simulink model "wing_landing_gear"  (R2015a)
settings: Solver=ode45  StartTime=0  StopTime=10  RelTol=1e-4  AbsTol=1e-4
model workspace (MAT data in the model file):
  grey = [0.5 0.5 0.5]
  lgrey = [0.7 0.7 0.7]
  dgrey = [0.3 0.3 0.3]
  ddgrey = [0.15 0.15 0.15]
  rho_alum = 2700
undefined symbols (not defined in the file): sigbuilder_block, X, Y, Z
libraries: sm_lib x59, sm_wing_landing_gear_lib x45, nesl_utility x7, simulink x2
(part 3 of 3)

== system wing_landing_gear/Wing Landing Gear/Main Column/Main Column/Spherical Cup and Holder/Cup ==
  Base-Center Transform : sm_lib/Frames and Transforms/Rigid Transform  TranslationMethod=StandardAxis  TranslationLengthUnit=cm  TranslationStandardAxis=+Z  TranslationStandardOffset=Ro  TranslationCartesianOffset=[0 0 0]  TranslationROffset=[]  TranslationROffsetUnits=m  TranslationZOffset=[]  TranslationZOffsetUnits=m  TranslationThetaOffset=[]  TranslationThetaOffsetUnits=deg  RotationMethod=None  RotationAngleUnits=deg  RotationStandardAxis=+X  RotationAngle=[]  RotationArbitraryAxis=[]  FollAlignAxisA=+X  BaseAlignAxisA=+Y  FollAlignAxisB=+Y  BaseAlignAxisB=+Z  RotationMatrix=[1 0 0; 0 1 0; 0 0 1]  BlockFunction=simmechanics.library.frames_transforms.rigid_transform
  Center-Strip A Transform : sm_lib/Frames and Transforms/Rigid Transform  TranslationMethod=None  TranslationLengthUnit=m  TranslationStandardAxis=+X  TranslationStandardOffset=0  TranslationCartesianOffset=[0 0 0]  TranslationROffset=[]  TranslationROffsetUnits=m  TranslationZOffset=[]  TranslationZOffsetUnits=m  TranslationThetaOffset=[]  TranslationThetaOffsetUnits=deg  RotationMethod=AlignedAxes  RotationAngleUnits=deg  RotationStandardAxis=+X  RotationAngle=[]  RotationArbitraryAxis=[]  FollAlignAxisA=+Y  BaseAlignAxisA=+Z  FollAlignAxisB=+Z  BaseAlignAxisB=-Y  RotationMatrix=[1 0 0; 0 1 0; 0 0 1]  BlockFunction=simmechanics.library.frames_transforms.rigid_transform
  Center-Strip B Transform : sm_lib/Frames and Transforms/Rigid Transform  TranslationMethod=None  TranslationLengthUnit=m  TranslationStandardAxis=+X  TranslationStandardOffset=0  TranslationCartesianOffset=[0 0 0]  TranslationROffset=[]  TranslationROffsetUnits=m  TranslationZOffset=[]  TranslationZOffsetUnits=m  TranslationThetaOffset=[]  TranslationThetaOffsetUnits=deg  RotationMethod=AlignedAxes  RotationAngleUnits=deg  RotationStandardAxis=+X  RotationAngle=[]  RotationArbitraryAxis=[]  FollAlignAxisA=+Z  BaseAlignAxisA=+X  FollAlignAxisB=+Y  BaseAlignAxisB=+Z  RotationMatrix=[1 0 0; 0 1 0; 0 0 1]  BlockFunction=simmechanics.library.frames_transforms.rigid_transform
  Cup Strip A : sm_lib/Body Elements/Solid  InertiaType=CalculateFromGeometry  Mass=[]  MassUnits=kg  CenterOfMass=[]  CenterOfMassUnits=m  MomentsOfInertia=[]  MomentsOfInertiaUnits=kg*m^2  ProductsOfInertia=[]  ProductsOfInertiaUnits=kg*m^2  DensityBased=on  Density=rho  DensityUnits=kg/(m^3)  GraphicType=FromGeometry  MarkerShape=Sphere  MarkerSize=10  MarkerSizeUnits=m  GraphicVisPropType=SimpleVisualProperties  GraphicDiffuseColor=Cc  GraphicSpecularColor=[0.8 0.8 0.8 1.0]  GraphicAmbientColor=[0.5 0.0 0.0 1.0]  GraphicEmissiveColor=[0.0 0.0 0.0 1.0]  GraphicShininess=64.0  GraphicOpacity=1  GeometryShape=GeneralExtrusion  RectangleSize=[]  RectangleSizeUnits=m  BrickDimensions=[]  BrickDimensionUnits=m  CylinderRadius=0.5  CylinderRadiusUnits=m  CylinderLength=1  CylinderLengthUnits=m  SphereRadius=0.5  SphereRadiusUnits=m  EllipsoidRadii=[]  EllipsoidRadiiUnits=m  ExtrusionCrossSection=cup_profile  ExtrusionCrossSectionUnits=cm  ExtrusionLength=T  ExtrusionLengthUnits=cm  PolygonNumSides=[]  PolygonOuterRadius=[]  PolygonOuterRadiusUnits=m  ExtGeomFileType=STL  ExtGeomFileUnits=m  RevolutionCrossSection=[1 1; 1 -1; 2 -1; 2 1]  RevolutionCrossSectionUnits=m  RevolutionExtent=Full  RevolutionAngle=180  RevolutionAngleUnits=deg  BlockFunction=simmechanics.library.body_elements.solid
  Cup Strip B : sm_lib/Body Elements/Solid  InertiaType=CalculateFromGeometry  Mass=[]  MassUnits=kg  CenterOfMass=[]  CenterOfMassUnits=m  MomentsOfInertia=[]  MomentsOfInertiaUnits=kg*m^2  ProductsOfInertia=[]  ProductsOfInertiaUnits=kg*m^2  DensityBased=on  Density=rho  DensityUnits=kg/(m^3)  GraphicType=FromGeometry  MarkerShape=Sphere  MarkerSize=10  MarkerSizeUnits=m  GraphicVisPropType=SimpleVisualProperties  GraphicDiffuseColor=Cc  GraphicSpecularColor=[0.8 0.8 0.8 1.0]  GraphicAmbientColor=[0.5 0.0 0.0 1.0]  GraphicEmissiveColor=[0.0 0.0 0.0 1.0]  GraphicShininess=64.0  GraphicOpacity=1  GeometryShape=GeneralExtrusion  RectangleSize=[]  RectangleSizeUnits=m  BrickDimensions=[]  BrickDimensionUnits=m  CylinderRadius=0.5  CylinderRadiusUnits=m  CylinderLength=1  CylinderLengthUnits=m  SphereRadius=0.5  SphereRadiusUnits=m  EllipsoidRadii=[]  EllipsoidRadiiUnits=m  ExtrusionCrossSection=cup_profile  ExtrusionCrossSectionUnits=cm  ExtrusionLength=T  ExtrusionLengthUnits=cm  PolygonNumSides=[]  PolygonOuterRadius=[]  PolygonOuterRadiusUnits=m  ExtGeomFileType=STL  ExtGeomFileUnits=m  RevolutionCrossSection=[1 1; 1 -1; 2 -1; 2 1]  RevolutionCrossSectionUnits=m  RevolutionExtent=Full  RevolutionAngle=180  RevolutionAngleUnits=deg  BlockFunction=simmechanics.library.body_elements.solid
  B : PMIOPort  Tag=PMCPort  Port=1  Side=Left
  C : PMIOPort  Tag=PMCPort  Port=2  Side=Right
  connections:
  B/RConn1 -- Base-Center Transform/LConn1
  Base-Center Transform/RConn1 -- Center-Strip A Transform/LConn1 -- Center-Strip B Transform/LConn1 -- C/RConn1
  Cup Strip A/RConn1 -- Center-Strip A Transform/RConn1
  Cup Strip B/RConn1 -- Center-Strip B Transform/RConn1
